simulink model "F16AltitudeAutopilotDesignSim"  (R2013a)
settings: Solver=ode45  StartTime=0.0  StopTime=100  RelTol=1e-3
values from neighbouring files (symbols this model uses):
  A = [0	393.72	0	-393.72	0	0 ... (first row only)    [F16AltitudeAutopilotDesign.m]    (also in F16AltitudeAutopilotDesign2.m = [0	393.72	0	-393.72	0	0	0; F16AltitudeAutopilotDesign2_addVilocity.m = [0	393.72	0	-393.72	0	0	0; F16AltitudeAutopilotDesign2_vhold.m = [0	393.72	0	-393.72	0	0	0; F16AltitudeAutopilotDesign_test.m = [0	393.72	0	-393.72	0	0	0)
  B = [0 ... (first row only)    [F16AltitudeAutopilotDesign.m]    (also in F16AltitudeAutopilotDesign2.m = [0	0; F16AltitudeAutopilotDesign2_addVilocity.m = [0	0; F16AltitudeAutopilotDesign2_vhold.m = [0	0; F16AltitudeAutopilotDesign_test.m = [0	0)
  C = [C_q;C_theta;C_h]    [F16AltitudeAutopilotDesign.m]    (also in F16AltitudeAutopilotDesign2.m = [0 0 0 57.29577951 0 0 0; F16AltitudeAutopilotDesign2_addVilocity.m = [0 0 0 57.29577951 0 0 0; F16AltitudeAutopilotDesign2_vhold.m = [0 0 0 57.29577951 0 0 0; F16AltitudeAutopilotDesign_test.m = [0 0 0 57.29577951 0 0 0)
  D = [0 ... (first row only)    [F16AltitudeAutopilotDesign.m]    (also in F16AltitudeAutopilotDesign2.m = [0	0; F16AltitudeAutopilotDesign2_addVilocity.m = [0	0; F16AltitudeAutopilotDesign2_vhold.m = [0	0; F16AltitudeAutopilotDesign_test.m = [0	0)
  k_alpha = 0.1    [F16AltitudeAutopilotDesign2.m]    (also in F16AltitudeAutopilotDesign2_addVilocity.m; F16AltitudeAutopilotDesign2_vhold.m; F16AltitudeAutopilotDesign_test.m = 0)
  k_ll = 0.6    [F16AltitudeAutopilotDesign2.m]    (also in F16AltitudeAutopilotDesign2_addVilocity.m; F16AltitudeAutopilotDesign2_vhold.m; F16AltitudeAutopilotDesign_test.m = 0.3)
  k_q = 2    [F16AltitudeAutopilotDesign.m]    (also in F16AltitudeAutopilotDesign2.m = 0.45; F16AltitudeAutopilotDesign2_addVilocity.m = 0.45; F16AltitudeAutopilotDesign2_vhold.m = 0.45; F16AltitudeAutopilotDesign_test.m = 0.5)
  kp = 1    [F16AltitudeAutopilotDesign2.m]    (also in F16AltitudeAutopilotDesign2_addVilocity.m; F16AltitudeAutopilotDesign2_vhold.m; F16AltitudeAutopilotDesign_test.m = 0.6)
  pole_l = 3    [F16AltitudeAutopilotDesign2.m]    (also in F16AltitudeAutopilotDesign2_addVilocity.m; F16AltitudeAutopilotDesign2_vhold.m; F16AltitudeAutopilotDesign_test.m)
  pole_p = 1    [F16AltitudeAutopilotDesign2.m]    (also in F16AltitudeAutopilotDesign2_addVilocity.m; F16AltitudeAutopilotDesign2_vhold.m; F16AltitudeAutopilotDesign_test.m)
libraries: simulink x1
settings Model: Creator=Dai  LastModifiedBy=Dai

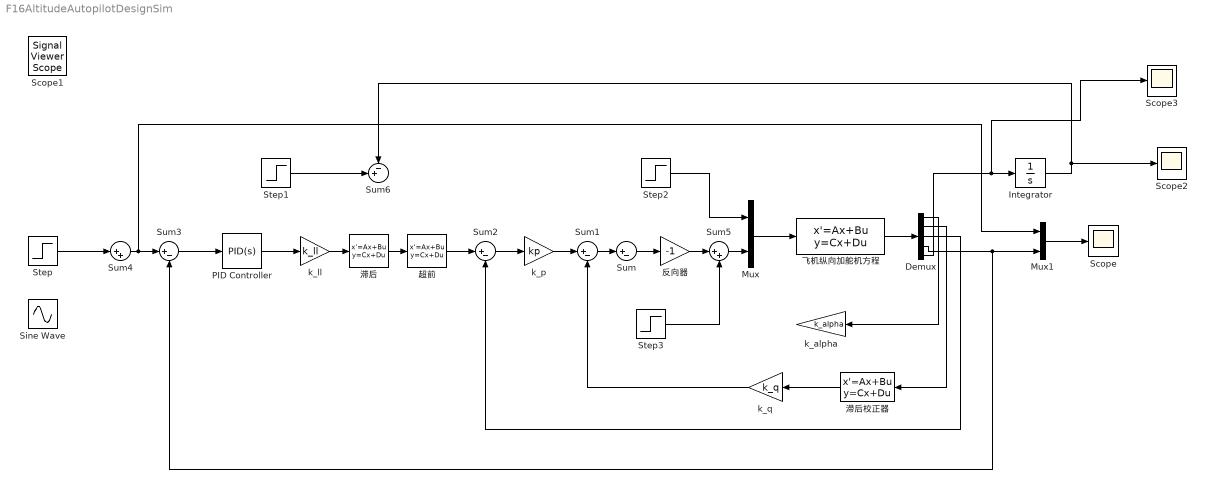
== system F16AltitudeAutopilotDesignSim ==
  Demux : Demux  Outputs=5
  Integrator : Integrator
  Mux : Mux  Inputs=2
  Mux1 : Mux  Inputs=2
  PID Controller : simulink/Continuous/PID Controller  Controller=PID  TimeDomain=Continuous-time  SampleTime=1  IntegratorMethod=Forward Euler  FilterMethod=Forward Euler  Form=Parallel  P=1  I=0.02  D=0  N=100  InitialConditionSource=internal  InitialConditionForIntegrator=0  InitialConditionForFilter=0  ExternalReset=none  LimitOutput=off  UpperSaturationLimit=inf  LowerSaturationLimit=-inf  LinearizeAsGain=on  AntiWindupMode=none  Kb=1  TrackingMode=off  Kt=1  PParamMin=[]  PParamMax=[]  IParamMin=[]  IParamMax=[]  DParamMin=[]  DParamMax=[]  NParamMin=[]  NParamMax=[]  KbParamMin=[]  KbParamMax=[]  KtParamMin=[]  KtParamMax=[]  POutMin=[]  POutMax=[]  IOutMin=[]  IOutMax=[]  DOutMin=[]  DOutMax=[]  NOutMin=[]  NOutMax=[]  KbOutMin=[]  KbOutMax=[]  KtOutMin=[]  KtOutMax=[]  IntegratorOutMin=[]  IntegratorOutMax=[]  FilterOutMin=[]  FilterOutMax=[]  SumOutMin=[]  SumOutMax=[]  SumI1OutMin=[]  SumI1OutMax=[]  SumI2OutMin=[]  SumI2OutMax=[]  SumI3OutMin=[]  SumI3OutMax=[]  SumDOutMin=[]  SumDOutMax=[]  SaturationOutMin=[]  SaturationOutMax=[]  IntegratorContinuousStateAttributes=''  IntegratorStateMustResolveToSignalObject=off  IntegratorRTWStateStorageClass=Auto  FilterContinuousStateAttributes=''  FilterStateMustResolveToSignalObject=off  FilterRTWStateStorageClass=Auto
  Scope : Scope
      settings: TimeRange=30  YMin=-0.5  YMax=3.5
  Scope2 : Scope
      settings: TimeRange=30  YMin=-0.5  YMax=3.5
  Scope3 : Scope
      settings: TimeRange=30  YMin=-0.5  YMax=3.5  SaveName=ScopeData2
  Sine Wave : Sin  Amplitude=0.5  Frequency=0.2  SampleTime=0
  Step : Step  Time=30  SampleTime=0  ZeroCross=off
  Step1 : Step  Time=20  After=10  SampleTime=0  ZeroCross=off
  Step2 : Step  Time=20  After=-6.6  SampleTime=0  ZeroCross=off
  Step3 : Step  Time=20  After=0.022  SampleTime=0  ZeroCross=off
  Sum{,1..3} (4 alike) : Sum  Inputs=|+-
  Sum4 : Sum  Inputs=|++
  Sum5 : Sum  Inputs=|++
  Sum6 : Sum  Inputs=-+|
  k_alpha : Gain  Gain=k_alpha
  k_ll : Gain  Gain=k_ll
  k_p : Gain  Gain=kp
  k_q : Gain  Gain=k_q
  反向器 : Gain  Gain=-1
  滞后 : StateSpace  A=-0.01  B=0.01  C=2
  滞后校正器 : StateSpace  A=-pole_p  C=zero_p-pole_p
  超前 : StateSpace  A=-pole_l  B=pole_l  C=-0.875
  飞机纵向加舵机方程 : StateSpace  A=A  B=B  C=C  D=D
  Scope1 : SignalViewerScope  IOType=viewer  RefreshTime=0.035000
  wires:
  Mux/1 -> 飞机纵向加舵机方程/1
  飞机纵向加舵机方程/1 -> Demux/1
  Demux/1 -> k_alpha/1
  Demux/2 -> 滞后校正器/1
  滞后校正器/1 -> k_q/1
  k_q/1 -> Sum1/2
  Sum1/1 -> Sum/1
  k_p/1 -> Sum1/1
  Demux/3 -> Sum2/2
  Sum2/1 -> k_p/1
  k_ll/1 -> 滞后/1
  滞后/1 -> 超前/1
  Demux/4 -> Mux1/2, Sum3/2
  Sum/1 -> 反向器/1
  PID Controller/1 -> k_ll/1
  Sum3/1 -> PID Controller/1
  Sum4/1 -> Mux1/1, Sum3/1
  Mux1/1 -> Scope/1
  Demux/5 -> Scope3/1, Integrator/1
  Integrator/1 -> Sum6/1, Scope2/1
  Step1/1 -> Sum6/2
  Step/1 -> Sum4/1
  超前/1 -> Sum2/1
  反向器/1 -> Sum5/1
  Sum5/1 -> Mux/2
  Step3/1 -> Sum5/2
  Step2/1 -> Mux/1
